simulink model "QueueOverWritingPolicyModel"  (R2019b)
settings: Solver=VariableStepAuto  StartTime=0.0  StopTime=10.0  RelTol=1e-3
undefined symbols (not defined in the file): m, n
libraries: simulink x1
settings Model: Creator=The MathWorks, Inc.  LastModifiedBy=The MathWorks, Inc.

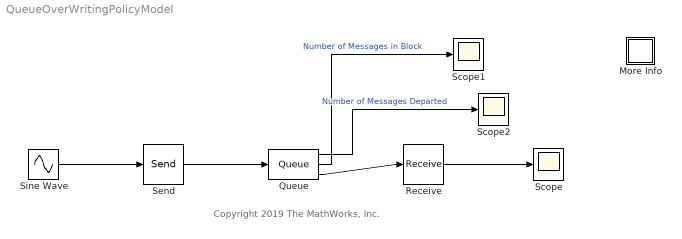
== system QueueOverWritingPolicyModel ==
  note: Copyright 2019 The MathWorks, Inc.
  More Info : Subsystem
      settings: OpenFcn=showExample('simulink/UseAQueueBlockToManageMessagesExample')
      mask Display: disp('?')
  Queue : Queue  InputPortMessageModes=m  OutputPortMessageModes=n,n,m  Capacity=16  NumberEntitiesDeparted=on  NumberEntitiesInBlock=on
      settings: OutputPortMap=o0,o1,o5
  Receive : Receive  InputPortMessageModes=m  UseInternalQueue=off  QueueOverwriting=on  QueueLength=1  QueueType=LIFO  SampleTime=0.1
  Scope : Scope
  Scope1 : Scope
  Scope2 : Scope
  Send : Send  OutputPortMessageModes=m
  Sine Wave : Sin  SampleTime=0.1
  wires:
  Queue/1 -> Scope2/1  "Number of Messages Departed"
  Receive/1 -> Scope/1
  Send/1 -> Queue/1
  Sine Wave/1 -> Send/1
  Queue/2 -> Scope1/1  "Number of Messages in Block"
  Queue/3 -> Receive/1

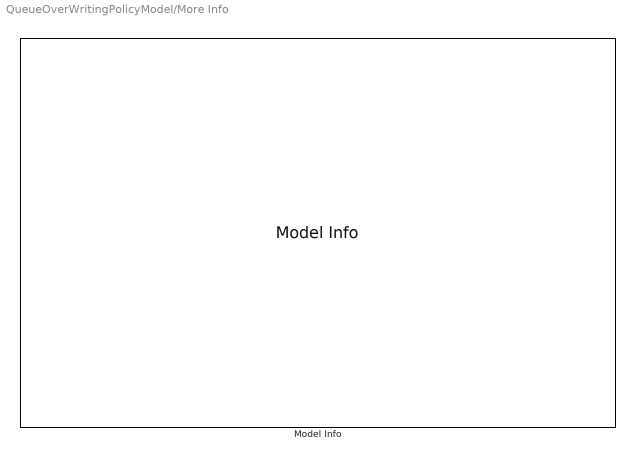
== system QueueOverWritingPolicyModel/More Info ==
  Model Info : simulink/Model-Wide Utilities/Model Info  Frame=on  DisplayStringWithTags=|  HorizontalTextAlignment=Left  LeftAlignmentValue=0.02
      | Model Description:
      | -------------------
      | This example shows how to use the Message Delay block to model a variable
      | speed conveyor belt between two airport terminals. The passengers step on
      | the conveyor belt following a Poisson distribution. Since passengers are
      | discrete entities, they are naturally modeled by Simulink(R) messages,
      | which are created by the Entity Generator block. When a passenger, i.e.,
      | a Simulink(R) message, is sent to the Message Delay block, the block
      | will hold it until it arrives at the other end of the conveyor belt. The
      | length of the delay time is automatically calculated by Simulink(R) based
      | on the ETA (estimated time of arrival), which is calculated by the
      | Stateflow(R) Chart. The operation of the conveyor belt depends on the
      | load and its transfer characteristics.
